simulink model "filtres"  (R2018a)
settings: Solver=VariableStepAuto  StartTime=0.0  StopTime=10.0  RelTol=1e-3
undefined symbols (not defined in the file or in its folder): den_band, den_high, den_low, num_band, num_high, num_low
libraries: dspsnks4 x1, dspvision x1
settings Model: Creator=cyrie  LastModifiedBy=cyrie

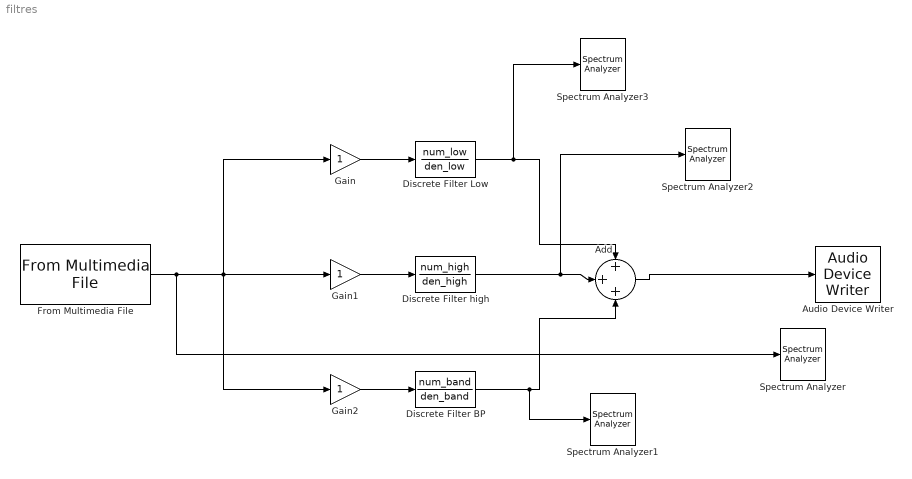
== system filtres ==
  Add : Sum  Inputs=+++
  Audio Device Writer : dspsnks4/Audio Device Writer  Driver=DirectSound  Device=Default  InheritSampleRate=on  SampleRate=44100  BitDepth=16-bit integer  BufferSize=4096  NumBuffers=10  DefaultOutputChannelMapping=on  OutputChannelMapping=1:2  OutputNumUnderrunSamples=off  DriverIdx=1  DeviceWarnFlag=''
  "Discrete Filter BP " : DiscreteFilter  Numerator=num_band  Denominator=den_band
  Discrete Filter Low : DiscreteFilter  Numerator=num_low  Denominator=den_low
  Discrete Filter high : DiscreteFilter  Numerator=num_high  Denominator=den_high
  From Multimedia File : dspvision/From Multimedia File  inputFilename=D:\A trier\Musique\Ludovico Einaudi -Essentiel\2. Una Mattina.mp3  loop=on  numPlays=inf  outputStreams=Audio only  videoDataType=single  audioDataType=double  inheritSampleTime=on  userDefinedSampleTime=1/30  noAudioOutput=off  isIntensityVideo=off  fourcc=RGB  colorVideoFormat=Separate color signals  outputEOF=off  dataOrg=Column-major  audioFrameSize=1024  computeAudioFrameSize=off  outSamplingMode=Sample based
      settings: SourceProductBaseCode=VP
  Gain : Gain
  Gain1 : Gain
  Gain2 : Gain
  Spectrum Analyzer{,1..3} (4 alike) : SpectrumAnalyzer
  wires:
  Gain2/1 -> "Discrete Filter BP "/1
  Gain1/1 -> Discrete Filter high/1
  Gain/1 -> Discrete Filter Low/1
  From Multimedia File/1 -> Spectrum Analyzer/1, Gain1/1, Gain/1, Gain2/1
  Add/1 -> Audio Device Writer/1
  Discrete Filter Low/1 -> Spectrum Analyzer3/1, Add/1
  Discrete Filter high/1 -> Spectrum Analyzer2/1, Add/2
  "Discrete Filter BP "/1 -> Spectrum Analyzer1/1, Add/3
